simulink model "PWM_Single_Phase_Inverter"  (R2025a)
settings: Solver=ode23tb  StartTime=0.0  StopTime=0.1  MaxStep=1e-4  RelTol=1e-3
libraries: spsIGBTDiodeLib x4, spsRMSLib x1, spsSeriesRLCBranchLib x1, spsVoltageMeasurementLib x1, spsDCVoltageSourceLib x1, sps_lib x1
settings Model: Creator=Jawad  LastModifiedBy=Jawad

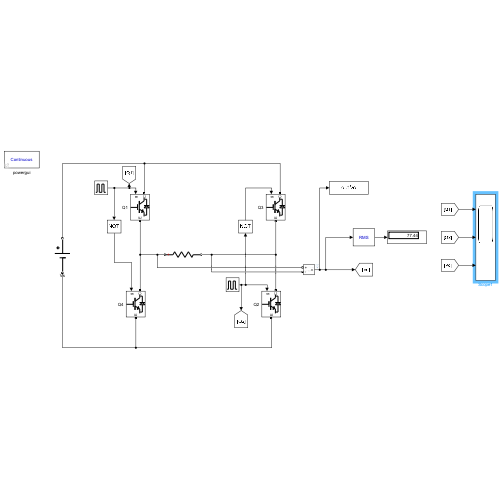
[thumbnail: Simulink's stored preview of the top-level diagram]
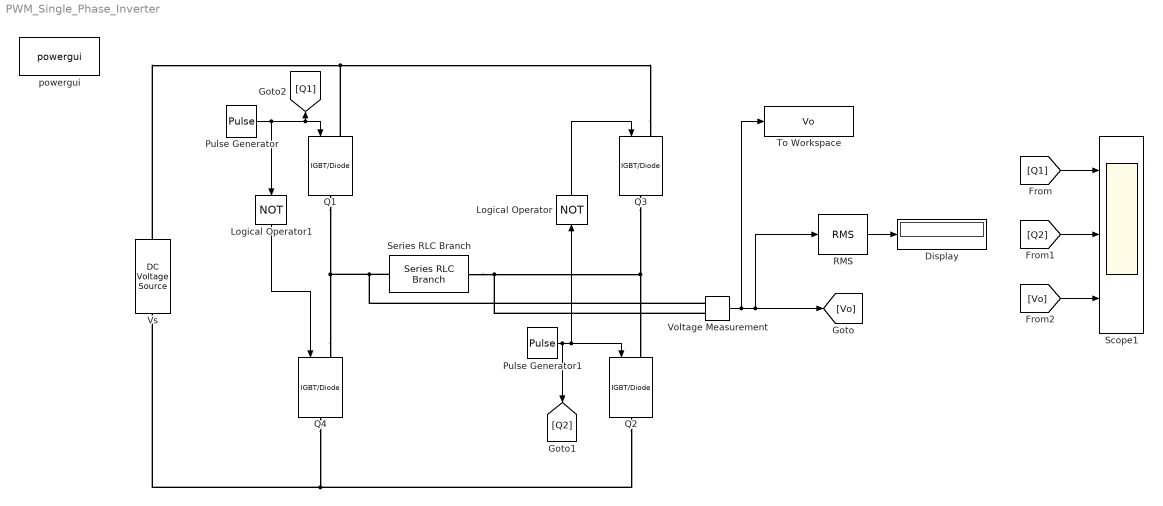
== system PWM_Single_Phase_Inverter ==
  Display : Display
  Logical Operator : Logic  Operator=NOT  AllPortsSameDT=off  OutDataTypeStr=boolean
  Logical Operator1 : Logic  Operator=NOT  AllPortsSameDT=off  OutDataTypeStr=boolean
  Pulse Generator : DiscretePulseGenerator  PulseType=Time based  Period=0.02  PulseWidth=50
  Pulse Generator1 : DiscretePulseGenerator  PulseType=Time based  Period=0.02  PulseWidth=50  PhaseDelay=90*(0.02/360)
  Q{1..4} (4 alike) : spsIGBTDiodeLib/IGBT//Diode  Ron=1e-3  Rs=1e5  Cs=inf  Measurements=off
  RMS : spsRMSLib/RMS  TrueRMS=on  Freq=60  RMSInit=120  Ts=0
  Scope1 : Scope  NumInputPorts=3
      settings: ActiveDisplayString=3  Title=Vo  ActiveDisplayYMinimum=-124.97500249999995  ActiveDisplayYMaximum=124.97500249999995
  Series RLC Branch : spsSeriesRLCBranchLib/Series RLC Branch  LConnTagsString=__new0  RConnTagsString=__new0  BranchType=R  Resistance=10  Inductance=1e-3  SetiL0=off  InitialCurrent=0  Capacitance=1e-6  Setx0=off  InitialVoltage=0  Measurements=None
  To Workspace : ToWorkspace  VariableName=Vo  SaveFormat=Structure With Time  SampleTime=-1
  Voltage Measurement : spsVoltageMeasurementLib/Voltage Measurement  PhasorSimulation=off  OutputType=Complex  PSBequivalent=0
  Vs : spsDCVoltageSourceLib/DC Voltage Source  Amplitude=100  Measurements=None
  powergui : sps_lib/powergui  Priority=1  SimulationMode=Continuous  SampleTime=50e-6  frequency=60  Iterations=50  frequencyindice=0  Pbase=100e6  ErrMax=1e-4  UnitsV=kV  UnitsW=MW  buscounter=0  FunctionMessages=off  echomessages=off  EnableUseOfTLC=off  CurrentSourceSwitches=off  DisableSnubberDevices=off  DisableRonSwitches=off  DisableVfSwitches=off  DisplayEquations=off  AutomaticDiscreteSolvers=off  SolverType=Tustin/Backward Euler (TBE)  Interpol=off  ExternalGateDelay=off  methode=off  Ts=100  x0status=blocks  SPID=on  SwTol=0  HookPort=off  NonlinearTolerance=1e-4  nMaxIteration=100  ContinueOnMaxIteration=off  RestoreLinks=warning  ResistiveCurrentMeasurement=off  Frange=[0:2:500]  Ylog=off  Xlog=on  ShowGrid=off  save=off  variable=ZData  structure=0  ZoomFFT=off  StartTime=0.0  cycles=1  DisplayStyle=1  fundamental=60  FreqAxis=off  MaxFrequency=1000  frequencyindicesteady=1  RmsSteady=1  display=off
  wires:
  RMS/1 -> Display/1
  Voltage Measurement/1 -> To Workspace/1, [Vo], RMS/1
  Pulse Generator/1 -> Logical Operator1/1, [Q1], Q1/1
  Pulse Generator1/1 -> Q2/1, Logical Operator/1, [Q2]
  Logical Operator/1 -> Q3/1
  Logical Operator1/1 -> Q4/1
  [Q1] -> Scope1/1
  [Vo] -> Scope1/3
  [Q2] -> Scope1/2
  connections:
  Q4/LConn1 -- Q1/RConn1 -- Voltage Measurement/LConn1 -- Series RLC Branch/LConn1
  Q3/LConn1 -- Vs/RConn1 -- Q1/LConn1
  Vs/LConn1 -- Q2/RConn1 -- Q4/RConn1
  Series RLC Branch/RConn1 -- Q3/RConn1 -- Q2/LConn1 -- Voltage Measurement/LConn2
